simulink subsystem "rail_constraints"  (R2024b)
settings: Solver=VariableStepAuto  StartTime=0.0  StopTime=10.0  RelTol=1e-3
undefined symbols (not defined in the file or in its folder): location, rail_length
settings Model: Creator=finnb  LastModifiedBy=finnb

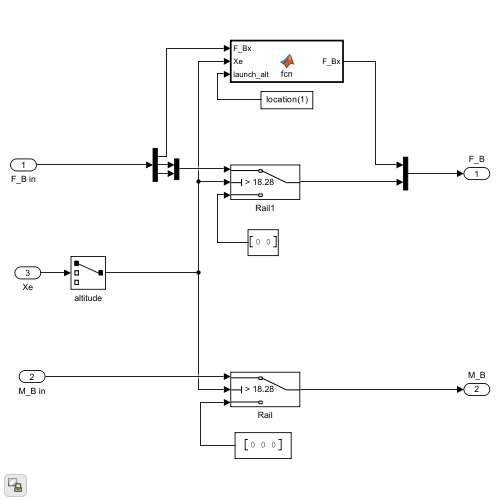
[thumbnail: Simulink's stored preview of the top-level diagram]
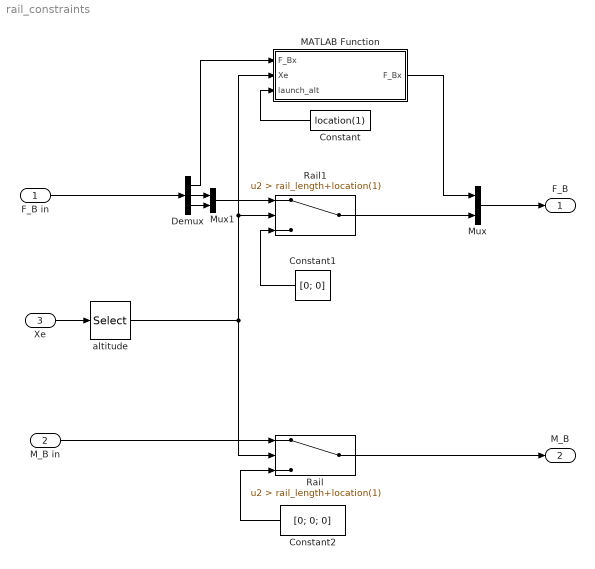
== system rail_constraints ==
  F_B in : Inport
  M_B in : Inport  Port=2
  Xe : Inport  Port=3
  Constant : Constant  Value=location(1)
  Constant1 : Constant  Value=[0; 0]
  Constant2 : Constant  Value=[0; 0; 0]
  Demux : Demux  Outputs=3
  MATLAB Function : MATLAB Function  TreatAsAtomicUnit=on
  Mux : Mux  Inputs=2
  Mux1 : Mux  Inputs=2
  Rail : Switch  Criteria=u2 > Threshold  Threshold=rail_length+location(1)  SaturateOnIntegerOverflow=off  InputSameDT=off
  Rail1 : Switch  Criteria=u2 > Threshold  Threshold=rail_length+location(1)  SaturateOnIntegerOverflow=off  InputSameDT=off
  altitude : Selector  InputPortWidth=3  IndexOptions=Index vector (dialog)  Indices=[1]  OutputSizes=1
  F_B : Outport  VectorParamsAs1DForOutWhenUnconnected=off
  M_B : Outport  Port=2  VectorParamsAs1DForOutWhenUnconnected=off
  wires:
  Demux/2 -> Mux1/1
  F_B in/1 -> Demux/1
  Mux1/1 -> Rail1/1
  Rail1/1 -> Mux/2
  Constant2/1 -> Rail/3
  Demux/1 -> MATLAB Function/1("F_Bx ")
  Xe/1 -> altitude/1
  Demux/3 -> Mux1/2
  Rail/1 -> M_B/1
  altitude/1 -> MATLAB Function/2(Xe), Rail1/2, Rail/2
  Mux/1 -> F_B/1
  Constant1/1 -> Rail1/3
  M_B in/1 -> Rail/1
  MATLAB Function/1(F_Bx) -> Mux/1
  Constant/1 -> MATLAB Function/3(launch_alt)

== matlab function rail_constraints/MATLAB Function ==
  data: F_Bx input; Xe input; F_Bx output; launch_alt input
function F_Bx = fcn(F_Bx, Xe, launch_alt)
   if Xe <= launch_alt
       if F_Bx <= 0
           F_Bx = 0;
       else
           return
       end
   else 
       return
   end
end
